simulink model "l1_lqr"  (R2025b)
settings: Solver=FixedStepAuto  StartTime=0.0  StopTime=10.0  RelTol=1e-3
undefined symbols (not defined in the file or in its folder): P
settings Model: Creator=eshikapathak  LastModifiedBy=eshikapathak

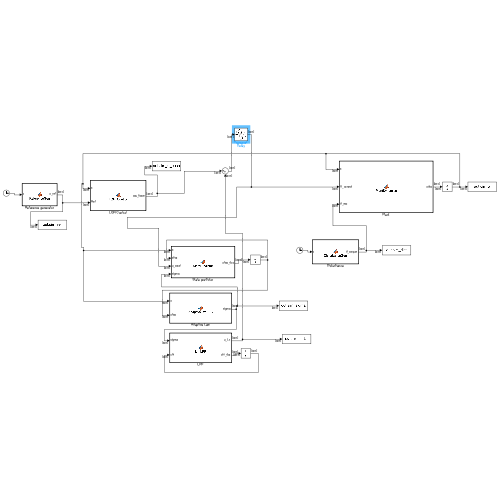
[thumbnail: Simulink's stored preview of the top-level diagram]
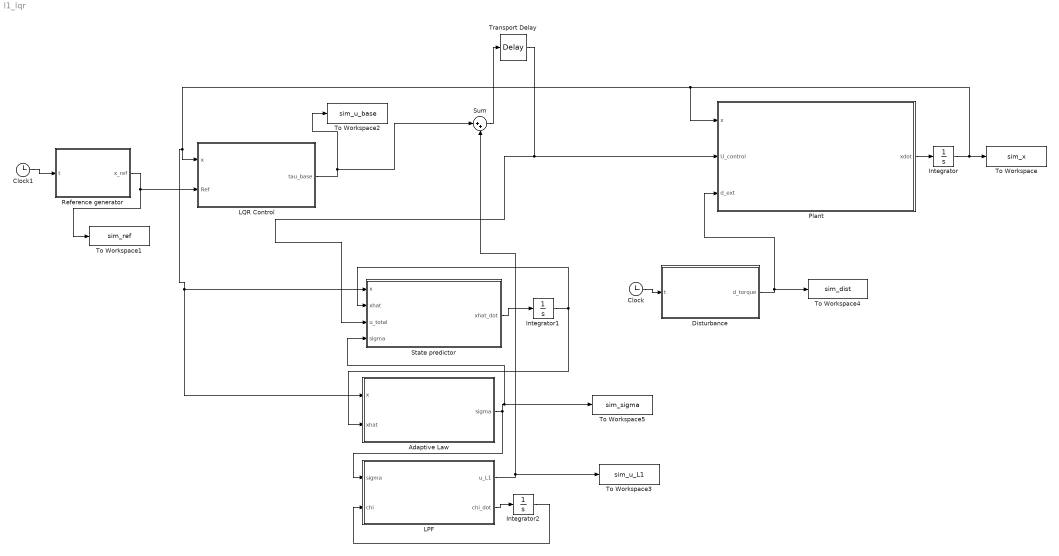
== system l1_lqr ==
  Adaptive Law : MATLAB Function  TreatAsAtomicUnit=on
  Clock : Clock
  Clock1 : Clock
  Disturbance : MATLAB Function  TreatAsAtomicUnit=on
  Integrator : Integrator
  Integrator1 : Integrator
  Integrator2 : Integrator
  LPF : MATLAB Function  TreatAsAtomicUnit=on
  LQR Control : MATLAB Function  TreatAsAtomicUnit=on
  Plant : MATLAB Function  TreatAsAtomicUnit=on
  Reference generator : MATLAB Function  TreatAsAtomicUnit=on
  State predictor : MATLAB Function  TreatAsAtomicUnit=on
  Sum : Sum  Inputs=|++
  To Workspace : ToWorkspace  VariableName=sim_x  SaveFormat=Timeseries  SampleTime=-1
  To Workspace1 : ToWorkspace  VariableName=sim_ref  SaveFormat=Timeseries  SampleTime=-1
  To Workspace2 : ToWorkspace  VariableName=sim_u_base  SaveFormat=Timeseries  SampleTime=-1
  To Workspace3 : ToWorkspace  VariableName=sim_u_L1  SaveFormat=Timeseries  SampleTime=-1
  To Workspace4 : ToWorkspace  VariableName=sim_dist  SaveFormat=Timeseries  SampleTime=-1
  To Workspace5 : ToWorkspace  VariableName=sim_sigma  SaveFormat=Timeseries  SampleTime=-1
  Transport Delay : TransportDelay  DelayTime=P.loop_delay  BufferSize=1000000
  wires:
  Plant/1(xdot) -> Integrator/1
  Integrator/1 -> To Workspace/1, Plant/1(x), LQR Control/1(x), Adaptive Law/1(x), State predictor/1(x)
  Reference generator/1(x_ref) -> LQR Control/2(Ref), To Workspace1/1
  Clock/1 -> Disturbance/1(t)
  Clock1/1 -> Reference generator/1(t)
  LQR Control/1(tau_base) -> To Workspace2/1, Sum/1
  LPF/1(u_L1) -> To Workspace3/1, Sum/2
  State predictor/1(xhat_dot) -> Integrator1/1
  Integrator1/1 -> Adaptive Law/2(xhat), State predictor/2(xhat)
  Adaptive Law/1(sigma) -> To Workspace5/1, State predictor/4(sigma), LPF/1(sigma)
  LPF/2(chi_dot) -> Integrator2/1
  Integrator2/1 -> LPF/2(chi)
  Transport Delay/1 -> Plant/2(U_control), State predictor/3(u_total)
  Disturbance/1(d_torque) -> To Workspace4/1, Plant/3(d_ext)
  Sum/1 -> Transport Delay/1

== matlab function l1_lqr/LQR Control ==
  data: x input; tau_base output size=[3 1]; Ref input; P parameter
function tau_base = LQR_Control(x, Ref, P)
    % Standard State Feedback
    error = x - Ref;
    tau_base = -P.K * error;
end

== matlab function l1_lqr/Plant ==
  data: x input; xdot output size=[6 1]; U_control input; d_ext input; P parameter
function xdot = PlantDynamics(x, U_control, d_ext, P)
    % Unpack parameters
    Ix = P.Ix; Iy = P.Iy; Iz = P.Iz; L = P.L;
    
    % States
    % x = [phi, theta, psi, p, q, r]
    p = x(4); q = x(5); r = x(6);
    
    % Total Torque = Control Input + External Disturbance
    % U_control is [U2(Roll), U3(Pitch), U4(Yaw)] 
    % Note: In your script U2/U3 were forces multiplied by L inside dynamics.
    % Let's standardize: Inputs to this block are TORQUES.
    
    tau_phi   = L * U_control(1) + d_ext(1);
    tau_theta = L * U_control(2) + d_ext(2);
    tau_psi   =     U_control(3) + d_ext(3); 
    
    % Rotational Dynamics (Euler Equations)
    p_dot = q*r*(Iy - Iz)/Ix + (1/Ix) * tau_phi;
    q_dot = p*r*(Iz - Ix)/Iy + (1/Iy) * tau_theta;
    r_dot = p*q*(Ix - Iy)/Iz + (1/Iz) * tau_psi;
    
    % Kinematics (Linearized mapping for simplicity, or use full rotation matrix)
    phi_dot   = p;
    theta_dot = q;
    psi_dot   = r;
    
    xdot = [phi_dot; theta_dot; psi_dot; p_dot; q_dot; r_dot];
end

== matlab function l1_lqr/State predictor ==
  data: x input; xhat_dot output size=[6 1]; xhat input; u_total input; sigma input; P parameter
function xhat_dot = StatePredictor(x, xhat, u_total, sigma, P)
    % Unpack sigma into Matched (m) and Unmatched (um)
    sigma_m  = sigma(1:3);
    sigma_um = sigma(4:6);
    
    xt = xhat - x;
    
    % Predictor Dynamics
    % xhat_dot = A*xhat + Bm*(u + sigma_m) + Bum*sigma_um + Ae*xt
    xhat_dot = P.A_true * xhat ...
             + P.Bm * (u_total + sigma_m) ...
             + P.Bum * sigma_um ...
             + P.Ae * xt;
end

== matlab function l1_lqr/Adaptive Law ==
  settings: updateMethod=DISCRETE  sampleTime=P.Ts
  data: x input; sigma output size=[6 1]; xhat input; P parameter
function sigma = AdaptiveLaw_PC(x, xhat, P)
    % Define persistent variables to hold sigma for the interval
    persistent sigma_hold
    if isempty(sigma_hold)
        sigma_hold = zeros(6,1);
    end
    
    % Error
    xt = xhat - x;
    
    % Calculations (Closed Form Piecewise Constant)
    % Phi = Ae^-1 * (exp(Ae*Ts) - I)
    % We calculate this dynamically or pass it in. 
    % For efficiency, perform this only once or pass pre-calcs in P.
    
    Phi = P.Ae \ (expm(P.Ae*P.Ts) - eye(6));
    E   = expm(P.Ae*P.Ts);
    
    % z = Phi^-1 * exp(Ae*Ts) * xt(k)
    z = Phi \ (E * xt);
    
    % Bbar * sigma = -z
    % Bbar is square (6x6) because it is [Bm Bum]
    Bbar = [P.Bm, P.Bum];
    
    sigma_new = -(Bbar \ z);
    
    sigma = sigma_new;
end

== matlab function l1_lqr/LPF ==
  data: sigma input; u_L1 output size=[3 1]; chi input; chi_dot output size=[3 1]; P parameter
function [u_L1, chi_dot] = L1_LPF(sigma, chi, P)
    % 1. Extract Matched Uncertainty
    % The LPF only filters the matched component (first 3 elements)
    sigma_m = sigma(1:3);
    
    % 2. Filter Dynamics (State Space)
    % chi_dot = Alpf * chi + Blpf * sigma_m
    chi_dot = P.Alpf * chi + P.Blpf * sigma_m;
    
    % 3. Calculate Control Signal
    % u_L1 = - (Clpf * chi) 
    % We apply the negative sign here to cancel the disturbance.
    % (Dlpf is zero in this design, so we skip it)
    
    u_L1 = -(P.Clpf * chi);
end

== matlab function l1_lqr/Reference generator ==
  data: t input; x_ref output size=[6 1]; P parameter
function x_ref = ReferenceGen(t, P)
    % desired angles [phi; theta; psi]
    % desired rates  [p; q; r]
    
    % Logic: Step input after t > P.ref_start
    if t >= P.ref_start
        ref_angles = [P.ref_amp; 0; 0];
    else
        ref_angles = [0; 0; 0];
    end
    
    ref_rates = [0; 0; 0];
    
    % Combine into full state reference
    x_ref = [ref_angles; ref_rates];
end

== matlab function l1_lqr/Disturbance ==
  data: t input; d_torque output size=[3 1]; P parameter
function d_torque = DisturbanceGen(t, P)
    % Generates disturbance torques (Nm) based on time
    
    d_phi   = P.dist_amp(1) * sin(P.dist_freq(1) * t);
    d_theta = P.dist_amp(2) * sin(P.dist_freq(2) * t);
    d_psi   = P.dist_amp(3) * sin(P.dist_freq(3) * t);
    
    d_torque = [d_phi; d_theta; d_psi];
end
